simulink model "Simple_Controller_SS_Model"  (R2022a)
settings: Solver=VariableStepAuto  StartTime=0.0  StopTime=0.001  RelTol=1e-3  AbsTol=1e-3
values from neighbouring files (symbols this model uses):
  den = cell2mat(den)    [FullBatteryControl.m]    (also in FullBatteryControl_SS_Model.m)
  LowerLimit = -CurrentLimit    [FullBatteryControl_SS_Model.m]
  num = cell2mat(num)    [FullBatteryControl.m]    (also in FullBatteryControl_SS_Model.m)
  SS_IC = SIM.SV_IC_Static    [FullBatteryControl_SS_Model.m]
  sys = multiple*ss(A,B,C,D)    [FullBatteryControl_SS_Model.m]
  UpperLimit = CurrentLimit    [FullBatteryControl_SS_Model.m]
undefined symbols (not defined in the file or in its folder): cell_voltage_0, den_sys, num_sys
settings Model: Creator=tyevans  LastModifiedBy=tyevans
settings DebuggingCC: UnconnectedInputMsg=warning  UnconnectedOutputMsg=warning  UnconnectedLineMsg=warning  SFMachineParentedDataDiag=warning
settings RTWCC: DLArmComputeVersion=19.05

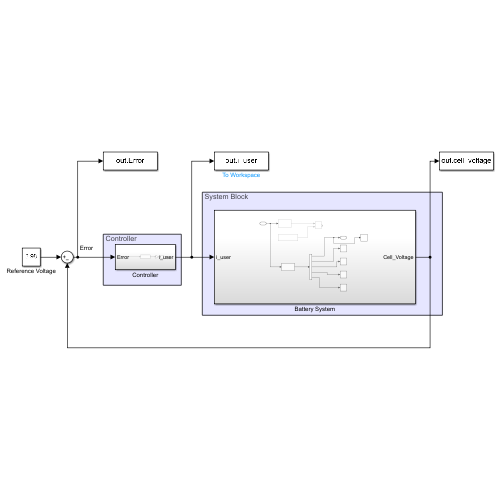
[thumbnail: Simulink's stored preview of the top-level diagram]
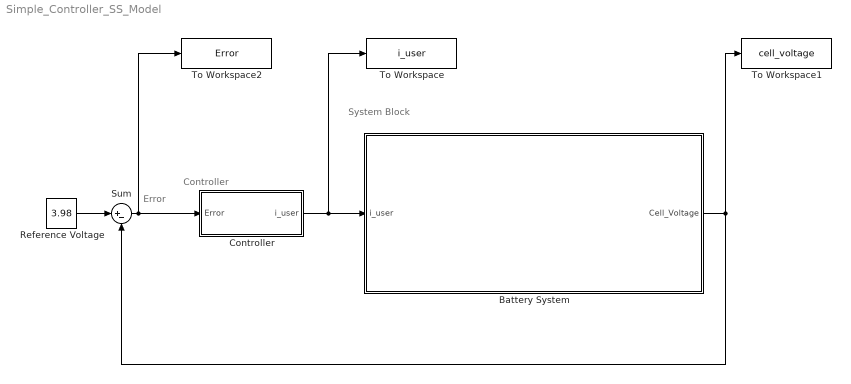
== system Simple_Controller_SS_Model ==
  note: Error
  note: System Block
  note: Controller
  Battery System : Subsystem
  Controller : Subsystem
  Reference Voltage : Constant  Value=3.98
  Sum : Sum  Inputs=|+-
  To Workspace : ToWorkspace  VariableName=i_user  SampleTime=-1
  To Workspace1 : ToWorkspace  VariableName=cell_voltage  SampleTime=-1
  To Workspace2 : ToWorkspace  VariableName=Error  SampleTime=-1
  wires:
  Reference Voltage/1 -> Sum/1
  Battery System/1(Cell_Voltage) -> Sum/2, To Workspace1/1
  Controller/1(i_user) -> To Workspace/1, Battery System/1(i_user)
  Sum/1 -> Controller/1(Error), To Workspace2/1

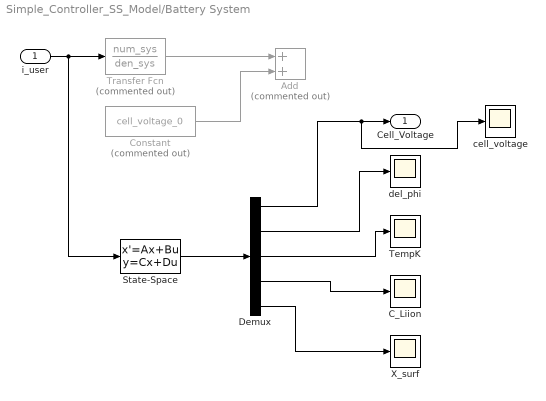
== system Simple_Controller_SS_Model/Battery System ==
  i_user : Inport
  Add : Sum  Commented=on
  C_Liion : Scope
  Constant : Constant  Commented=on  Value=cell_voltage_0
  Demux : Demux  Outputs=5
  State-Space : StateSpace  A=sys.A  B=sys.B  C=sys.C  D=sys.D  InitialCondition=SS_IC
  TempK : Scope
  Transfer Fcn : TransferFcn  Commented=on  Numerator=num_sys  Denominator=den_sys
  X_surf : Scope
  cell_voltage : Scope
  del_phi : Scope
  Cell_Voltage : Outport
  wires:
  i_user/1 -> State-Space/1, Transfer Fcn/1
  Transfer Fcn/1 -> Add/1
  Constant/1 -> Add/2
  State-Space/1 -> Demux/1
  Demux/1 -> cell_voltage/1, Cell_Voltage/1
  Demux/2 -> del_phi/1
  Demux/3 -> TempK/1
  Demux/4 -> C_Liion/1
  Demux/5 -> X_surf/1

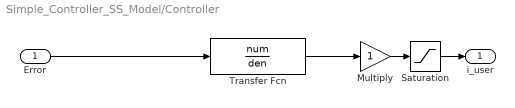
== system Simple_Controller_SS_Model/Controller ==
  Error : Inport
  Multiply : Gain
  Saturation : Saturate  UpperLimit=UpperLimit  LowerLimit=LowerLimit
  Transfer Fcn : TransferFcn  Numerator=num  Denominator=den
  i_user : Outport
  wires:
  Transfer Fcn/1 -> Multiply/1
  Error/1 -> Transfer Fcn/1
  Multiply/1 -> Saturation/1
  Saturation/1 -> i_user/1
